simulink model "SimuEchantSignalErr"  (Simulink 8.3)
settings: Solver=ode45  StartTime=0.0  StopTime=10  MaxStep=1e-2  RelTol=1e-3
values from neighbouring files (symbols this model uses):
  Te = [1 0.1 0.5 2 3]    [Simu.m]
libraries: cstblocks x6, simulink x2
settings Model: Creator=cadenat  LastModifiedBy=2asri13
settings OptimizationCC: ExpressionDepthLimit=2147483647
settings DebuggingCC: FcnCallInpInsideContextMsg=UseLocalSettings

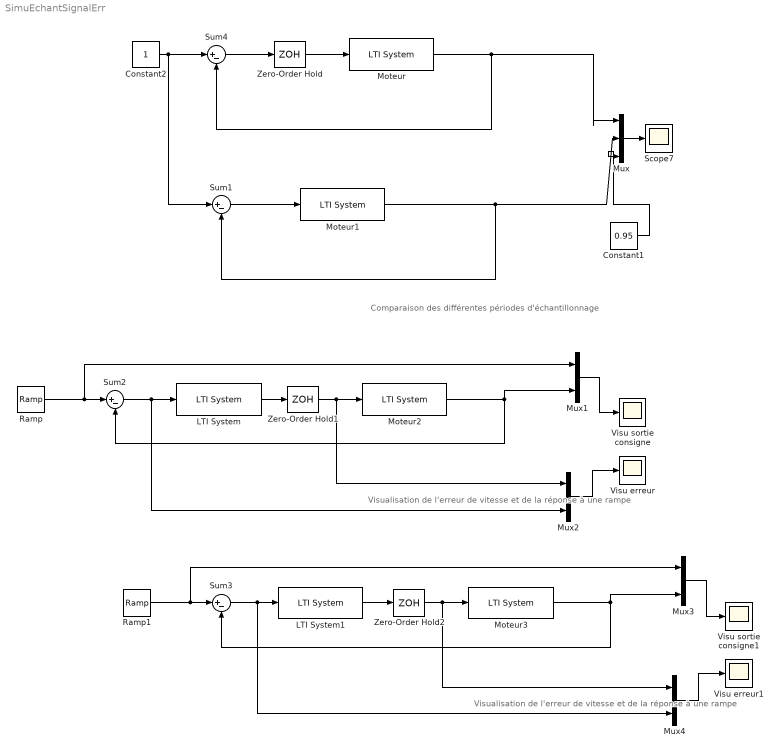
== system SimuEchantSignalErr ==
  note: Visualisation de l'erreur de vitesse et de la réponse à une rampe
  note: Comparaison des différentes périodes d'échantillonnage
  note: Visualisation de l'erreur de vitesse et de la réponse à une rampe
  Constant1 : Constant  Value=0.95
  Constant2 : Constant
  LTI System : cstblocks/LTI System  sys=Cp  IC=[]
  LTI System1 : cstblocks/LTI System  sys=C1  IC=[]
  Moteur{,1..3} (4 alike) : cstblocks/LTI System  sys=G  IC=[]
  Mux : Mux  Inputs=3
  Mux{1..4} (4 alike) : Mux  Inputs=2
  Ramp : simulink/Sources/Ramp  slope=1  start=0  X0=0
  Ramp1 : simulink/Sources/Ramp  slope=1  start=0  X0=0
  Scope7 : Scope
  Sum{1..4} (4 alike) : Sum  Inputs=|+-  SaturateOnIntegerOverflow=on  InputSameDT=on  OutDataTypeStr=Inherit: Same as first input
  Visu erreur : Scope
      settings: SaveName=ScopeData2
  Visu erreur1 : Scope
      settings: SaveName=ScopeData3
  Visu sortie consigne : Scope
  Visu sortie consigne1 : Scope
      settings: SaveName=ScopeData4
  Zero-Order Hold : ZeroOrderHold  SampleTime=Te(2)
  Zero-Order Hold1 : ZeroOrderHold  SampleTime=Te(2)
  Zero-Order Hold2 : ZeroOrderHold  SampleTime=Te(2)
  wires:
  Moteur/1 -> Sum4/2, Mux/1
  Constant2/1 -> Sum4/1, Sum1/1
  Sum4/1 -> Zero-Order Hold/1
  Zero-Order Hold/1 -> Moteur/1
  Sum1/1 -> Moteur1/1
  Moteur1/1 -> Sum1/2, Mux/2
  Mux/1 -> Scope7/1
  Moteur2/1 -> Sum2/2, Mux1/2
  Ramp/1 -> Sum2/1, Mux1/1
  Sum2/1 -> Mux2/2, LTI System/1
  Zero-Order Hold1/1 -> Moteur2/1, Mux2/1
  Mux1/1 -> Visu sortie consigne/1
  Mux2/1 -> Visu erreur/1
  Constant1/1 -> Mux/3
  LTI System/1 -> Zero-Order Hold1/1
  Moteur3/1 -> Sum3/2, Mux3/2
  Ramp1/1 -> Sum3/1, Mux3/1
  Sum3/1 -> LTI System1/1, Mux4/2
  Zero-Order Hold2/1 -> Moteur3/1, Mux4/1
  Mux3/1 -> Visu sortie consigne1/1
  Mux4/1 -> Visu erreur1/1
  LTI System1/1 -> Zero-Order Hold2/1
